simulink model "psi_w_new_model"  (R2017a)
settings: Solver=VariableStepAuto  StartTime=0.0  StopTime=10000  RelTol=1e-3
undefined symbols (not defined in the file or in its folder): Kw_wavegen, lambda_wavegen, w0_wavegen
libraries: simulink x1
settings Model: Creator=sondrna  LastModifiedBy=sondrna

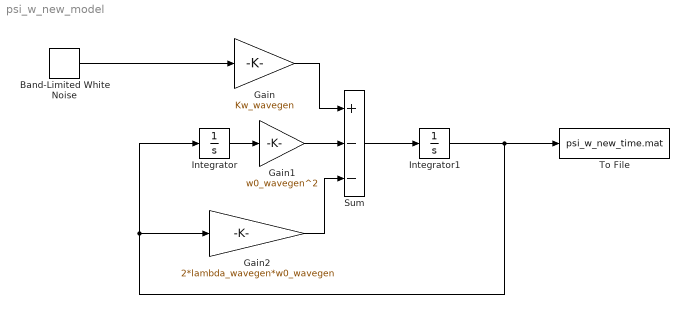
== system psi_w_new_model ==
  Band-Limited White Noise : simulink/Sources/Band-Limited White Noise  Cov=[1]  Ts=0.1  seed=[23341]
  Gain : Gain  Gain=Kw_wavegen
  Gain1 : Gain  Gain=w0_wavegen^2
  Gain2 : Gain  Gain=2*lambda_wavegen*w0_wavegen
  Integrator : Integrator
  Integrator1 : Integrator
  Sum : Sum  Inputs=+--
  To File : ToFile  Filename=psi_w_new_time.mat  MatrixName=psi_w
  wires:
  Integrator1/1 -> Gain2/1, Integrator/1, To File/1
  Sum/1 -> Integrator1/1
  Band-Limited White Noise/1 -> Gain/1
  Gain/1 -> Sum/1
  Integrator/1 -> Gain1/1
  Gain1/1 -> Sum/2
  Gain2/1 -> Sum/3
